simulink model "qss_example_cvtctrl"  (Simulink 6.6)
settings: Solver=VariableStepDiscrete  StartTime=0.0  StopTime=1220  RelTol=1e-3
undefined symbols (not defined in the file): g, h, P_CVT_opt, r_wheel, rho, w_CVT_opt
libraries: qss_tb_library x5
settings Model: Creator=csu  LastModifiedBy=csu  ExtModeAutoUpdateStatusClock=off
settings OptimizationCC: InlineInvariantSignals=on
settings DebuggingCC: SignalResolutionControl=TryResolveAllWithWarning  MultiTaskDSMMsg=warning  MultiTaskCondExecSysMsg=none  StrictBusMsg=None
settings RTWCC: IncludeERTFirstTime=on

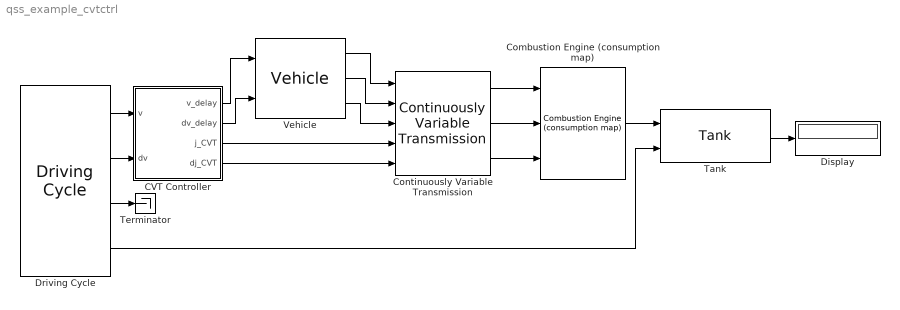
== system qss_example_cvtctrl ==
  CVT Controller : Subsystem  Tag=cvt controller  AncestorBlock=qss_tb_library/Controller/CVT Controller  mask(CVT Controller){j_CVT_min=3, j_CVT_max=15, w_wheel_min=3, w_CVT_idle=100, w_CVT_upper=300}
      mask prompts: j_CVT_min "Lower gear ratio limit [-]"; j_CVT_max "Upper gear ratio limit [-]"; w_wheel_min "Minimum wheel speed [rad/s]"; w_CVT_idle "CVT idle speed [rad/s]"; w_CVT_upper "Maximum CVT speed [rad/s]"
      mask help:
      | This block calculates the optimum gear ratio and its change during one integration step for a CVT.
      |
      | Input:
      | =====
      | 	v		Speed [m/s]
      | 	dv		Acceleration [m/s^2]
      |
      | Output:
      | ======
      | 	v_delay		Speed one step delayed [m/s]
      | 	dv_delay	Acceleration one step delayed [m/s^2]
      | 	j_CVT		Gear ratio [-]
      | 	dj_CVT		Change of gear ratio [1/s]
      mask init:
      | init_CVT_ctrl;
  Combustion Engine (consumption map) : qss_tb_library/Energy Converter/Combustion Engine (consumption map)  Tag=combustion engine  SystemSampleTime=-1  engine_type=Otto  V_d=0.708  scale_CE=1  theta_CE=0.05  w_CE_idle=105  P_CE_idle=2600  P_aux=300  ENABLE_FUEL_CUTOFF=on  T_CE_cutoff=-5  P_CE_cutoff=0
  Continuously Variable Transmission : qss_tb_library/Gear System/Continuously Variable Transmission  Tag=cvt  SystemSampleTime=-1  e_CVT=0.97  P_CVT0=400  w_wheel_min=3
  Display : Display
  Driving Cycle : qss_tb_library/Driving Cycle/Driving Cycle  Tag=cycle  SystemSampleTime=-1  cyclenr=Europe: NEDC  stepsize=1  autostop=on
  Tank : qss_tb_library/Energy Source/Tank  Tag=tank  SystemSampleTime=-1  fuel=Gasoline  flag_cold_start=on
  Terminator : Terminator
  Vehicle : qss_tb_library/Vehicle/Vehicle  Tag=vehicle  SystemSampleTime=-1  m_f=750  mt2m_f=5  A_f=1.8  d_wheel=0.5  cw=0.22  mu=0.008
  wires:
  Continuously Variable Transmission/1 -> Combustion Engine (consumption map)/1
  Continuously Variable Transmission/2 -> Combustion Engine (consumption map)/2
  Continuously Variable Transmission/3 -> Combustion Engine (consumption map)/3
  Tank/1 -> Display/1
  Combustion Engine (consumption map)/1 -> Tank/1
  Vehicle/1 -> Continuously Variable Transmission/1
  Vehicle/2 -> Continuously Variable Transmission/2
  Driving Cycle/1 -> CVT Controller/1(v)
  Driving Cycle/2 -> CVT Controller/2(dv)
  CVT Controller/1(v_delay) -> Vehicle/1
  CVT Controller/2(dv_delay) -> Vehicle/2
  Vehicle/3 -> Continuously Variable Transmission/3
  CVT Controller/3(j_CVT) -> Continuously Variable Transmission/4
  CVT Controller/4(dj_CVT) -> Continuously Variable Transmission/5
  Driving Cycle/4 -> Tank/2
  Driving Cycle/3 -> Terminator/1

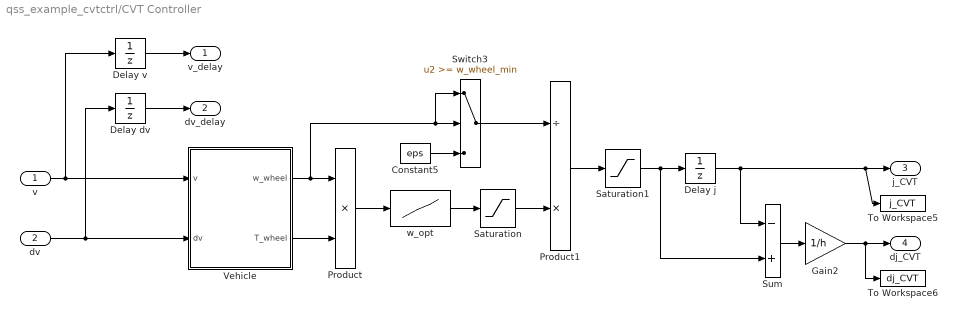
== system qss_example_cvtctrl/CVT Controller ==
  v : Inport
  dv : Inport  Port=2
  Constant5 : Constant  Value=eps
  Delay dv : UnitDelay  SampleTime=h
  Delay j : UnitDelay  X0=j_CVT_min  SampleTime=h
  Delay v : UnitDelay  SampleTime=h
  Gain2 : Gain  Gain=1/h  SaturateOnIntegerOverflow=on
  Product : Product  SaturateOnIntegerOverflow=on  RndMeth=Zero  InputSameDT=on
  Product1 : Product  Inputs=/*  SaturateOnIntegerOverflow=on  RndMeth=Zero  InputSameDT=on
  Saturation : Saturate  UpperLimit=w_CVT_upper  LowerLimit=w_CVT_idle
  Saturation1 : Saturate  UpperLimit=j_CVT_max  LowerLimit=j_CVT_min
  Sum : Sum  Inputs=-+  SaturateOnIntegerOverflow=on  InputSameDT=on
  Switch3 : Switch  Threshold=w_wheel_min  SaturateOnIntegerOverflow=on  InputSameDT=on
  To Workspace5 : ToWorkspace  VariableName=j_CVT  SampleTime=-1  SaveFormat=Array
  To Workspace6 : ToWorkspace  VariableName=dj_CVT  SampleTime=-1  SaveFormat=Array
  Vehicle : Subsystem  Tag=vehicle  AncestorBlock=qss_tb_library/Vehicle/Vehicle  mask(Vehicle){m_f=750, mt2m_f=5, A_f=1.8, d_wheel=0.5, cw=0.22, mu=0.008}
      mask prompts: m_f "Total mass of the vehicle [kg]"; mt2m_f "Rotating mass [%]"; A_f "Vehicle cross section [m^2]"; d_wheel "Wheel diameter [m]"; cw "Drag coefficient [-]"; mu "Rolling friction coefficient [-]"
      mask help:
      | This block computes the power required from the vehicle.
      |
      | Input:
      | =====
      | 	v		Speed [m/s]
      | 	dv		Acceleration [m/s^2]
      |
      | Output:
      | ======
      | 	w_wheel	Speed of the wheel [rad/s]
      | 	dw_wheel	Acceleration of the wheel [rad/s^2]
      | 	T_wheel	Torque on the wheel [Nm]
      mask init:
      | init_vehicle;
  w_opt : Lookup  InputValues=P_CVT_opt  OutputValues=w_CVT_opt  SaturateOnIntegerOverflow=on
  v_delay : Outport  InitialOutput=0
  dv_delay : Outport  Port=2  InitialOutput=0
  j_CVT : Outport  Port=3  InitialOutput=0
  dj_CVT : Outport  Port=4  InitialOutput=0
  wires:
  Sum/1 -> Gain2/1
  Delay v/1 -> v_delay/1
  w_opt/1 -> Saturation/1
  Product/1 -> w_opt/1
  Saturation1/1 -> Sum/2, Delay j/1
  Delay j/1 -> Sum/1, j_CVT/1, To Workspace5/1
  Switch3/1 -> Product1/1
  Delay dv/1 -> dv_delay/1
  v/1 -> Delay v/1, Vehicle/1(v)
  dv/1 -> Delay dv/1, Vehicle/2(dv)
  Constant5/1 -> Switch3/3
  Vehicle/1(w_wheel) -> Product/1, Switch3/1, Switch3/2
  Saturation/1 -> Product1/2
  Product1/1 -> Saturation1/1
  Vehicle/2(T_wheel) -> Product/2
  Gain2/1 -> dj_CVT/1, To Workspace6/1

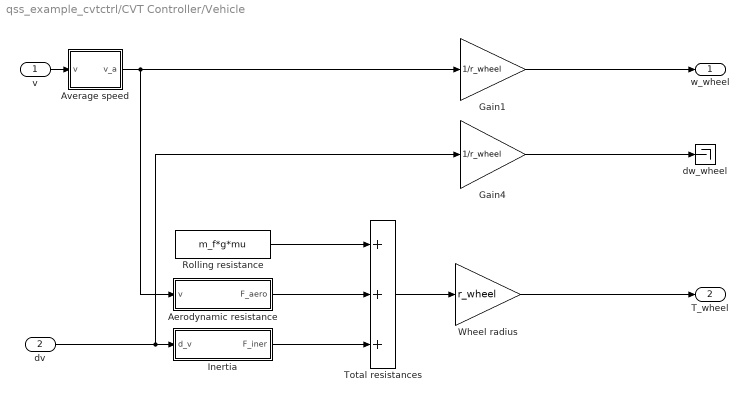
== system qss_example_cvtctrl/CVT Controller/Vehicle ==
  v : Inport
  dv : Inport  Port=2
  Aerodynamic resistance : Subsystem
  Average speed : Subsystem
  Gain1 : Gain  Gain=1/r_wheel  SaturateOnIntegerOverflow=on
  Gain4 : Gain  Gain=1/r_wheel  SaturateOnIntegerOverflow=on
  Inertia : Subsystem
  Rolling resistance : Constant  Value=m_f*g*mu
  Total resistances : Sum  Inputs=+++  SaturateOnIntegerOverflow=on  InputSameDT=on
  Wheel radius : Gain  Gain=r_wheel  SaturateOnIntegerOverflow=on
  dw_wheel : Terminator
  w_wheel : Outport  InitialOutput=0
  T_wheel : Outport  Port=2  InitialOutput=0
  wires:
  v/1 -> Average speed/1(v)
  dv/1 -> Gain4/1, Inertia/1(d_v)
  Average speed/1(v_a) -> Gain1/1, Aerodynamic resistance/1(v)
  Wheel radius/1 -> T_wheel/1
  Total resistances/1 -> Wheel radius/1
  Inertia/1(F_iner) -> Total resistances/3
  Aerodynamic resistance/1(F_aero) -> Total resistances/2
  Rolling resistance/1 -> Total resistances/1
  Gain1/1 -> w_wheel/1
  Gain4/1 -> dw_wheel/1

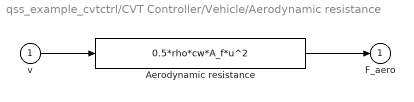
== system qss_example_cvtctrl/CVT Controller/Vehicle/Aerodynamic resistance ==
  v : Inport
  Aerodynamic resistance : Fcn  Expr=0.5*rho*cw*A_f*u^2
  F_aero : Outport  InitialOutput=0
  wires:
  Aerodynamic resistance/1 -> F_aero/1
  v/1 -> Aerodynamic resistance/1

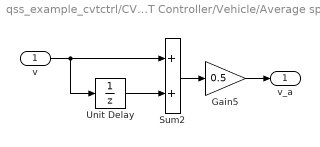
== system qss_example_cvtctrl/CVT Controller/Vehicle/Average speed ==
  v : Inport
  Gain5 : Gain  Gain=0.5  SaturateOnIntegerOverflow=on
  Sum2 : Sum  SaturateOnIntegerOverflow=on  InputSameDT=on
  Unit Delay : UnitDelay  SampleTime=h
  v_a : Outport  InitialOutput=0
  wires:
  v/1 -> Unit Delay/1, Sum2/1
  Gain5/1 -> v_a/1
  Sum2/1 -> Gain5/1
  Unit Delay/1 -> Sum2/2

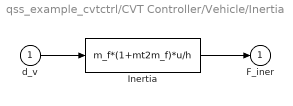
== system qss_example_cvtctrl/CVT Controller/Vehicle/Inertia ==
  d_v : Inport
  Inertia : Fcn  Expr=m_f*(1+mt2m_f)*u/h
  F_iner : Outport  InitialOutput=0
  wires:
  d_v/1 -> Inertia/1
  Inertia/1 -> F_iner/1
